simulink model "Servo_model_n"  (R2022b)
settings: Solver=ode5  StartTime=0.0  StopTime=5  FixedStep=0.01  RelTol=1e-3  AbsTol=1e-6
PreLoadFcn:
  | load servo_chstat
undefined symbols (not defined in the file or in its folder): pwm, vpwm
settings Model: ExtModeTrigDuration=12000  ExtModeTrigLevel=0.400000  Creator=jims  LastModifiedBy=artur
settings SolverCC: AutoScaleAbsTol=off  AlgebraicLoopSolver=TrustRegion
settings DataIOCC: ExternalInput=[]  InitialState=[]  MaxDataPoints=5000  SaveFormat=Array  SignalLoggingSaveFormat=ModelDataLogs  SaveOutput=off  SaveTime=off  ReturnWorkspaceOutputs=off  SignalLoggingName=sigsOut
settings OptimizationCC: BooleanDataType=off  ExpressionDepthLimit=2147483647  LifeSpan=inf
settings DebuggingCC: SaveWithParameterizedLinksMsg=none  UnderspecifiedInitializationDetection=Classic  MergeDetectMultiDrivingBlocksExec=none  SignalResolutionControl=TryResolveAllWithWarning  MultiTaskDSMMsg=warning  MultiTaskCondExecSysMsg=none  IntegerOverflowMsg=none  FcnCallInpInsideContextMsg=warning  UnconnectedInputMsg=warning  UnconnectedOutputMsg=warning  UnconnectedLineMsg=warning  AllowSymbolicDim=off  StateNameClashWarn=warning  PregeneratedLibrarySubsystemCodeDiagnostic=none  SFUnexpectedBacktrackingDiag=warning  SFNoUnconditionalDefaultTransitionDiag=warning  SFExecutionAtInitializationDiag=none  SFMachineParentedDataDiag=warning  IntegerSaturationMsg=none  ArithmeticOperatorsInVariantConditions=warning
settings HardwareCC: ProdBitPerLong=64  ProdHWDeviceType=Intel->x86-64 (Linux 64)  TargetBitPerLong=64  TargetBitPerPointer=64  TargetIntDivRoundTo=Zero  TargetEndianess=LittleEndian  TargetWordSize=64  TargetHWDeviceType=Intel->x86-64
settings ModelReferenceCC: EnableRefExpFcnMdlSchedulingChecks=on  PropagateSignalLabelsOutOfModel=off
settings SFSimCC: SimUseLocalCustomCode=off  CustomCodeUndefinedFunction=UseInterfaceOnly
settings RTWCC: Description=Simulink Desktop Real-Time  SystemTargetFile=sldrt.tlc  TemplateMakefile=sldrt.tmf  RTWUseLocalCustomCode=off  RTWCompilerOptimization=on
settings CodeAppCC: MaxIdLength=95  StateflowObjectComments=on
settings SimulinkDesktopRealTimeCC: TargetLibSuffix=_sldrt.a  TargetPreCompLibLocation=C:\Program Files\MATLAB\R2022b\toolbox\sldrt\lib\win64  TargetLangStandard=C89/C90 (ANSI)  SupportVariableSizeSignals=off
settings ConfigComp: CovMetricSettings=dw  CovSaveCumulativeToWorkspaceVar=on  CovSaveSingleToWorkspaceVar=on  CovExternalEMLEnable=off

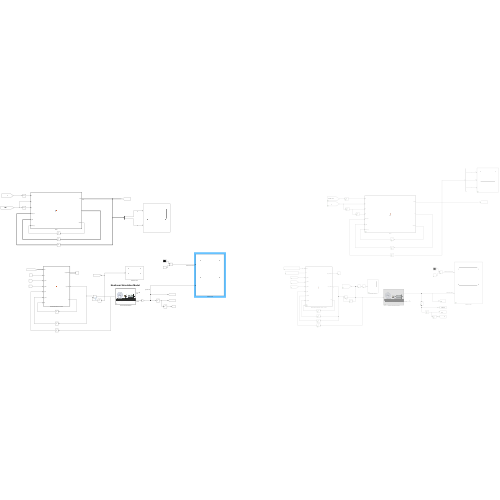
[thumbnail: Simulink's stored preview of the top-level diagram]
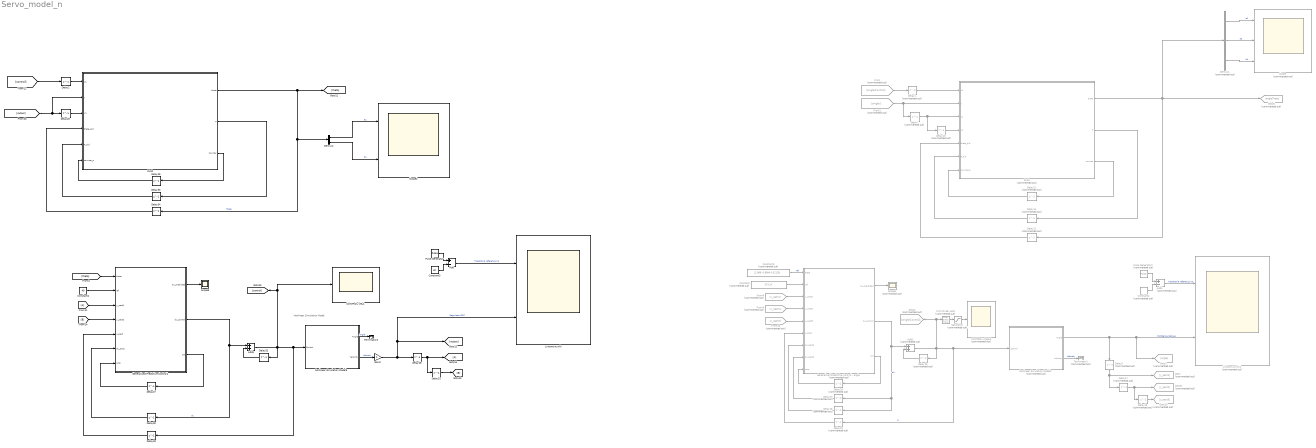
== system Servo_model_n ==
  note: Nonlinear Simulation Model
  Add : Sum  Inputs=+-
  Add2 : Sum  Commented=on
  Add3 : Sum
  Add4 : Sum  Commented=on  Inputs=+-
  CONTROL ANGLE : Scope  Commented=on
  CONTROL VEL1 : Scope
  Constant : Constant  Commented=on  Value=2*3.14
  Constant2 : Constant  Value=40
  Constant3 : Constant  Value=40
  Constant4 : Constant  Commented=on  Value=2*3.14
  Constant6 : Constant  Commented=on  Value=[1.988 -0.9884 0.01129]
  Delay1 : Delay  Commented=on  InitialCondition=0
  Delay{3,7,10,15..19} (8 alike) : Delay  Commented=on  DelayLength=1  InitialCondition=0
  Delay12 : Delay  Commented=on  DelayLength=1  InitialCondition=[2 -1 0.01]
  Delay14 : Delay  Commented=on  DelayLength=1  InitialCondition=eye(3) * 10^6
  Delay{2,25,28..32} (7 alike) : Delay  DelayLength=1  InitialCondition=0
  Delay20 : Delay  Commented=on  InitialCondition=0
  Delay21 : Delay  Commented=on  DelayLength=1  InitialCondition=10
  Delay24 : Delay  Commented=on  DelayLength=1  InitialCondition=1
  Delay26 : Delay  DelayLength=1  InitialCondition=10
  Delay27 : Delay  DelayLength=1  InitialCondition=1
  Delay33 : Delay  DelayLength=1  InitialCondition=eye(2) * 10^6
  Delay34 : Delay  DelayLength=1  InitialCondition=[0.79 1.9048]
  Demux1 : Demux  Commented=on  Outputs=3
  Demux2 : Demux  Outputs=2
  First Order Hold : FirstOrderHold  Commented=on  ErrorTolerance=inf
  From : From  Commented=on  GotoTag=angleControl
  From1 : From  Commented=on  GotoTag=angle
  From10 : From  Commented=on  GotoTag=y_past3
  From11 : From
  From8 : From  Commented=on  GotoTag=y_past1
  From9 : From  Commented=on  GotoTag=y_past2
  Gain2 : Gain
  Generalized Predictive Control - angle : MATLAB Function  Commented=on  TreatAsAtomicUnit=on
  Generalized Predictive Control1 : MATLAB Function  TreatAsAtomicUnit=on
  Goto : Goto  Commented=on  GotoTag=y_past1
  Goto1 : Goto  Commented=on  GotoTag=angle
  Goto10 : Goto  Commented=on  GotoTag=y_past3
  Goto14 : Goto
  Goto2 : Goto  Commented=on  GotoTag=angleControl
  Goto5 : Goto  Commented=on  GotoTag=angleTheta
  Goto9 : Goto  Commented=on  GotoTag=y_past2
  Liniowe wyniki : Scope  NumInputPorts=2
  Liniowe wyniki1 : Scope  Commented=on  NumInputPorts=2
  Nonlinear Simulation Model2 : Subsystem  Commented=on  mask{x0=[0 0], c_n=206, Parameter3=[vpwm pwm]}
      mask prompts: x0 "Initial conditions [angle velocity]"; c_n "Gain c"; Parameter3 "Static characteristic [velocity control]"
      mask Help:
      | The parameters necessary for this block are:
      | 1. Static characteristic implemented as Look-up table block (vectors vpwm and pwm),
      | 2. gain  - c ,
      | 3. Initial conditions - x0,
      | Refer to 3.2 section in User's Manual.
      | 
      | 
      | The model preloads the default static characteristic from servo_chstat.mat file.
      | To change default characteristic a user should load a new vpwm and pwm vectors or
      | replace servo_chstat.mat file.
      mask Display: image(imread('Servo_m.JPG'))
  Nonlinear Simulation Model3 : Subsystem  mask{x0=[0 0], c_n=206, Parameter3=[vpwm pwm]}
      mask prompts: x0 "Initial conditions [angle velocity]"; c_n "Gain c"; Parameter3 "Static characteristic [velocity control]"
      mask Help:
      | The parameters necessary for this block are:
      | 1. Static characteristic implemented as Look-up table block (vectors vpwm and pwm),
      | 2. gain  - c ,
      | 3. Initial conditions - x0,
      | Refer to 3.2 section in User's Manual.
      | 
      | 
      | The model preloads the default static characteristic from servo_chstat.mat file.
      | To change default characteristic a user should load a new vpwm and pwm vectors or
      | replace servo_chstat.mat file.
      mask Display: image(imread('Servo_m.JPG'))
  Pulse Generator : DiscretePulseGenerator  PulseType=Time based  Amplitude=80  Period=4  PulseWidth=50
  Pulse Generator2 : DiscretePulseGenerator  Commented=on  PulseType=Time based  Amplitude=4*pi  Period=4  PulseWidth=50
  RLS1 : MATLAB Function  Commented=on  TreatAsAtomicUnit=on
  RLS2 : MATLAB Function  TreatAsAtomicUnit=on
  Saturation : Saturate  Commented=on  UpperLimit=1  LowerLimit=-1
  Scope : Scope  Commented=on  NumInputPorts=3
  Scope2 : Scope  NumInputPorts=2
  Scope4 : Scope  Commented=on
  Scope5 : Scope
  Terminator1 : Terminator  Commented=on
  Terminator2 : Terminator
  wires:
  Gain2/1 -> Delay28/1, [output], Liniowe wyniki/2  "Regulator GPC"
  Delay30/1 -> Generalized Predictive Control1/6(du_past)
  [control] -> Delay2/1
  RLS2/1(theta) -> Demux2/1, Delay34/1, [theta]  "theta"
  Generalized Predictive Control1/1(du_predicted) -> Scope5/1
  Delay34/1 -> RLS2/4(theta_old)
  Delay33/1 -> RLS2/5(P_old)
  [output] -> Delay25/1, RLS2/2(y)
  Nonlinear Simulation Model3/1(Angle) -> Terminator2/1  "Angle"
  Demux2/2 -> Scope2/2  "b1"
  Nonlinear Simulation Model3/2(Velocity) -> Gain2/1  "Velocity"
  [B] -> Generalized Predictive Control1/4(y_past2)
  [theta] -> Generalized Predictive Control1/1(theta)
  Delay28/1 -> Delay31/1, Goto14/1
  Delay25/1 -> RLS2/3(y1)
  Add3/1 -> CONTROL VEL1/1, [control], Nonlinear Simulation Model3/1(Control), Delay29/1, Delay32/1
  From11/1 -> Generalized Predictive Control1/3(y_past1)
  Delay26/1 -> RLS2/6(counter_p)
  Delay29/1 -> Generalized Predictive Control1/5(u_past)
  Constant3/1 -> Add/2
  Constant2/1 -> Generalized Predictive Control1/2(ref)
  Pulse Generator/1 -> Add/1
  Generalized Predictive Control1/3(cnt) -> Delay27/1
  Add/1 -> Liniowe wyniki/1  "Trajektoria referencyjna"
  Delay32/1 -> Add3/2
  Delay27/1 -> Generalized Predictive Control1/7(cntp)
  RLS2/3(counter) -> Delay26/1
  Delay2/1 -> RLS2/1(u1)
  Generalized Predictive Control1/2(du_control) -> Delay30/1, Add3/1  "du"
  Delay31/1 -> [B]
  Demux2/1 -> Scope2/1  "a1"
  RLS2/2(P) -> Delay33/1
  From9/1 -> Generalized Predictive Control - angle/4(y_past2)
  From10/1 -> Generalized Predictive Control - angle/5(y_past3)
  Constant4/1 -> Add4/2
  Nonlinear Simulation Model2/1(Angle) -> Delay3/1, Liniowe wyniki1/2, Goto1/1  "Położenie kątowe"
  RLS1/1(theta) -> Delay12/1, Goto5/1, Demux1/1
  Delay3/1 -> Delay17/1, Goto/1
  Saturation/1 -> CONTROL ANGLE/1
  First Order Hold/1 -> Saturation/1
  Generalized Predictive Control - angle/3(cnt) -> Delay24/1
  Delay18/1 -> Goto10/1
  Delay19/1 -> Generalized Predictive Control - angle/6(u_past)
  Delay21/1 -> RLS1/7(counter_p)
  RLS1/3(counter) -> Delay21/1
  Pulse Generator2/1 -> Add4/1
  Generalized Predictive Control - angle/2(du_control) -> Delay16/1, Delay20/1, Add2/1  "du"
  Constant/1 -> Generalized Predictive Control - angle/2(ref)
  Constant6/1 -> Generalized Predictive Control - angle/1(theta)  "ref"
  From1/1 -> Delay7/1, RLS1/2(y)
  Delay24/1 -> Generalized Predictive Control - angle/9(cntp)
  From8/1 -> Generalized Predictive Control - angle/3(y_past1)
  Demux1/2 -> Scope/2  "a2"
  Demux1/3 -> Scope/3  "b1"
  Nonlinear Simulation Model2/2(Velocity) -> Terminator1/1  "Velocity"
  Add4/1 -> Liniowe wyniki1/1  "Trajektoria referencyjna"
  RLS1/2(P) -> Delay14/1
  Delay15/1 -> Add2/2
  Delay10/1 -> RLS1/4(y2)
  Generalized Predictive Control - angle/1(du_predicted) -> Scope4/1
  Delay16/1 -> Generalized Predictive Control - angle/7(du_past1)
  Delay14/1 -> RLS1/6(P_old)
  Delay7/1 -> Delay10/1, RLS1/3(y1)
  From/1 -> Delay1/1
  Delay1/1 -> RLS1/1(u2)
  Delay12/1 -> RLS1/5(theta_old)
  Add2/1 -> First Order Hold/1, Goto2/1, Delay15/1, Nonlinear Simulation Model2/1(Control), Delay19/1  "S"
  Delay17/1 -> Delay18/1, Goto9/1
  Delay20/1 -> Generalized Predictive Control - angle/8(du_past2)
  Demux1/1 -> Scope/1  "a1"

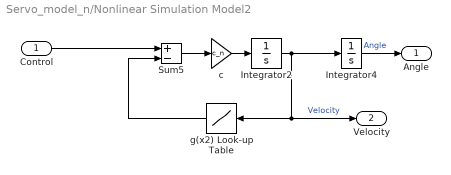
== system Servo_model_n/Nonlinear Simulation Model2 ==
  Control : Inport
  Integrator2 : Integrator  InitialCondition=x0(2)
  Integrator4 : Integrator  InitialCondition=x0(1)
  Sum5 : Sum  Inputs=+-  InputSameDT=on  SaturateOnIntegerOverflow=on  OutDataTypeStr=Inherit: Same as first input
  c : Gain  Gain=c_n  SaturateOnIntegerOverflow=on  OutDataTypeStr=Inherit: Same as input  ParamDataTypeStr=Inherit: Same as input
  g(x2) Look-up Table : Lookup  InputValues=vpwm  Table=pwm
  Angle : Outport  InitialOutput=0  VectorParamsAs1DForOutWhenUnconnected=off
  Velocity : Outport  Port=2  InitialOutput=0  VectorParamsAs1DForOutWhenUnconnected=off
  wires:
  Control/1 -> Sum5/1
  c/1 -> Integrator2/1
  Integrator4/1 -> Angle/1  "Angle"
  Integrator2/1 -> g(x2) Look-up Table/1, Velocity/1, Integrator4/1  "Velocity"
  g(x2) Look-up Table/1 -> Sum5/2
  Sum5/1 -> c/1

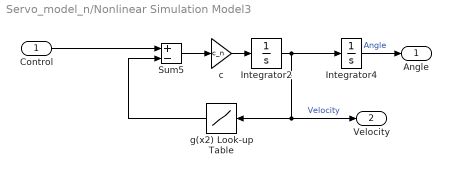
== system Servo_model_n/Nonlinear Simulation Model3 ==
  Control : Inport
  Integrator2 : Integrator  InitialCondition=x0(2)
  Integrator4 : Integrator  InitialCondition=x0(1)
  Sum5 : Sum  Inputs=+-  InputSameDT=on  SaturateOnIntegerOverflow=on  OutDataTypeStr=Inherit: Same as first input
  c : Gain  Gain=c_n  SaturateOnIntegerOverflow=on  OutDataTypeStr=Inherit: Same as input  ParamDataTypeStr=Inherit: Same as input
  g(x2) Look-up Table : Lookup  InputValues=vpwm  Table=pwm
  Angle : Outport  InitialOutput=0  VectorParamsAs1DForOutWhenUnconnected=off
  Velocity : Outport  Port=2  InitialOutput=0  VectorParamsAs1DForOutWhenUnconnected=off
  wires:
  Control/1 -> Sum5/1
  c/1 -> Integrator2/1
  Integrator4/1 -> Angle/1  "Angle"
  Integrator2/1 -> g(x2) Look-up Table/1, Velocity/1, Integrator4/1  "Velocity"
  g(x2) Look-up Table/1 -> Sum5/2
  Sum5/1 -> c/1

== matlab function Servo_model_n/RLS1 ==
  data: u2 input; y input; y1 input; y2 input; theta output; theta_old input; P_old input; P output; counter_p input; counter output
function [theta,P,counter]= fcn(u2,y,y1,y2,theta_old,P_old,counter_p)

counter = counter_p;

lambda = 0.985;

phi = [y1;y2;u2];

if counter_p == 10

K = P_old * phi/(lambda + phi'*P_old*phi);

P = ((eye(3) - K * phi') * P_old) * lambda^-1;

theta = theta_old + K * (y - phi'*theta_old);

counter = 0;
else

theta = theta_old;
P = P_old;
counter = counter + 1;
end

== matlab function Servo_model_n/Generalized Predictive Control - angle ==
  data: du_predicted output; theta input; ref input; y_past1 input; y_past2 input; y_past3 input; u_past input; du_past1 input; du_control output; du_past2 input; cnt output; cntp input
function [du_predicted, du_control,cnt] = fcn(theta,ref,y_past1,y_past2,y_past3,u_past,du_past1,du_past2,cntp)

cnt = cntp;

%Współczynniki modelu z algorytmu RLS
a1 = -theta(1);
a2 = -theta(2);
b1 = theta(3);

%Parametry
ny = 32; %HORYZONT PREDYKCJI
nu = 8; %HORYZONT STEROWANIA
lambda = 1.2;

%Przeszłe wyjścia
y_past = [y_past1;y_past2;y_past3];
du_past = [du_past1;du_past2];

%Trajektoria referencyjna, stała

%%% trajektoria referencyjna
Ts = 0.01; %PRÓBKOWANIE SYMULACJI
sim_time = 4; %CZAS SYMULACJI

traj_ub = ref*ones(1/Ts*sim_time/2,1);

traj_lb = -ref*ones(1/Ts*sim_time/2,1);


trajektoria = [traj_ub;traj_lb;traj_ub];

ref = trajektoria(cnt:ny+cnt-1, 1);

cnt = cntp + 1;

if cnt == 30*100-ny
    cnt = 1;
end

%%%

%Czy wykorzystać T-filtr?
filtrowanie = false;

%Ograniczenia
%true - ograniczenia na y, false - bez ograniczeń na y
ograniczenie_wyjscia = true;

du_max = 1;
du_min = -1;
u_max = 1;
u_min = -1;
y_max = 6.6;
y_min = -6.6;

%Wyznaczenie wielomianów a i b
a = [1 a1 a2];
b = [0 0 b1];
A = conv(a,[1 -1]);

%Wyznaczenie macierzy predykcji
[Ca,Ha] = predmat(A,ny);
[Cb,Hb] = predmat(b,ny);

Cai = inv(Ca);

H = Cai*Cb;
P = Cai*Hb;
Q = Cai*(-Ha);

%%%%%%%%%%%%%%%%%%%%%%%%%%%%%%%%%%%%%%%%%%%%%%%%%%%%%%%%%%%%%%%%%%%%%%%%%%%

if filtrowanie == true
    Tfilt = [1 -0.05];
    
    [Ct,Ht] = predmat(Tfilt,ny);
    Pfilt = Ct * P - H * Ht;
    Qfilt = Ct * Q + Ht;
    
    P = Pfilt;
    Q = Qfilt;
end

%%%%%%%%%%%%%%%%%%%%%%%%%%%%%%%%%%%%%%%%%%%%%%%%%%%%%%%%%%%%%%%%%%%%%%%%%%%

Hu = H(:,1:nu); %horyzont sterowania

%Ustawienie ograniczeń dla optymalizatora 

%Prawo sterowania dla algorytmu z ograniczeniami
S = Hu'*Hu + eye(nu)*lambda;
S = (S + S')/2;
f = Hu'*Q * y_past + Hu'*P * du_past - Hu' * ref;

    if ograniczenie_wyjscia == true
        %OGRANICZENIA Z Y
        [C,dd,du,ddu,dy] = mpc_ograniczenia(du_max, du_min,u_max,u_min,y_max,y_min,nu,Hu,P,Q,2,3);
        dt = dd + du * u_past + ddu * du_past + dy*y_past;
    else
        %OGRANICZENIA BEZ Y
        [C, dd,du] = mpc_ograniczenia_bez_y(du_max,du_min,u_max,u_min,nu);
        dt = dd + du * u_past;
    end


opts = optimoptions('quadprog','Algorithm','active-set');

x0 = 0.1*eye(nu,1);

du_predicted = quadprog(S,f,C,dt,[],[],[],[],x0,opts);

du_control = du_predicted(1);

%Prawo sterowania dla algorytmu bez ograniczeń
% Pr = ( inv(Hu'*Hu+lambda*eye(nu)) ) * Hu';
% Nk = Pr*Q;
% Dk = Pr*P;
% 
% du_predicted = Pr * ref - Dk * du_past - Nk*y_past;
% du_control = du_predicted(1);

== matlab function Servo_model_n/Generalized Predictive Control1 ==
  data: du_predicted output; theta input; ref input; y_past1 input; y_past2 input; u_past input; du_past input; du_control output; cntp input; cnt output
function [du_predicted, du_control,cnt] = fcn(theta,ref,y_past1,y_past2,u_past,du_past,cntp)

cnt = cntp;

%Współczynniki modelu z algorytmu RLS
a1 = -theta(1);
b1 = theta(2);

%Przeszłe wyjścia
y_past = [y_past1;y_past2];
    
%Parametry
ny = 32; %HORYZONT PREDYKCJI
nu = 12; %HORYZONT STEROWANIA
lambda = 0.5;
    
%Czy wykorzystać T-filtr?
filtrowanie = false;
    
%Ograniczenia
%true - ograniczenia na y, false - bez ograniczeń na y
ograniczenie_wyjscia = true;

du_max = 1;
du_min = -1;
u_max = 1;
u_min = -1;
y_max = 42;
y_min = -42;

%Trajektoria referencyjna, stała
Ts = 0.01; %PRÓBKOWANIE SYMULACJI
sim_time = 4; %CZAS SYMULACJI

traj_ub = ref*ones(1/Ts*sim_time/2,1);

traj_lb = -ref*ones(1/Ts*sim_time/2,1);

%%% trajektoria referencyjna
trajektoria = [traj_ub;traj_lb;traj_ub;-ref*ones(ny,1)];

ref = trajektoria(cnt:ny+cnt-1, 1);

cnt = cntp + 1;

%%%



    %Wyznaczenie wielomianów a i b
    a = [1 a1];
    b = [0 b1];
    A = conv(a,[1 -1]);
    
    %Wyznaczenie macierzy predykcji
    [Ca,Ha] = predmat(A,ny);
    [Cb,Hb] = predmat(b,ny);
    
    Cai = inv(Ca);
    
    H = Cai*Cb;
    P = Cai*Hb;
    Q = Cai*(-Ha);

%%%%%%%%%%%%%%%%%%%%%%%%%%%%%%%%%%%%%%%%%%%%%%%%%%%%%%%%%%%%%%%%%%%%%%%%%%%

if filtrowanie == true
    Tfilt = [1 -0.2];
    
    [Ct,Ht] = predmat(Tfilt,ny);
    Pfilt = Ct * P - H * Ht;
    Qfilt = Ct * Q + Ht;
    
    P = Pfilt;
    Q = Qfilt;
end

%%%%%%%%%%%%%%%%%%%%%%%%%%%%%%%%%%%%%%%%%%%%%%%%%%%%%%%%%%%%%%%%%%%%%%%%%%%

    Hu = H(:,1:nu); %horyzont sterowania

%Ustawienie ograniczeń dla optymalizatora 

%Prawo sterowania dla algorytmu z ograniczeniami
    S = Hu'*Hu + eye(nu)*lambda;
    S = (S + S')/2;
    f = Hu'*Q * y_past + Hu'*P * du_past - Hu' * ref;

    if ograniczenie_wyjscia == true
        %OGRANICZENIA Z Y
        [C,dd,du,ddu,dy] = mpc_ograniczenia(du_max, du_min,u_max,u_min,y_max,y_min,nu,Hu,P,Q,1,2);
        dt = dd + du * u_past + ddu * du_past + dy*y_past;
    else
        %OGRANICZENIA BEZ Y
        [C, dd,du] = mpc_ograniczenia_bez_y(du_max,du_min,u_max,u_min,nu);
        dt = dd + du * u_past;
    end


    opts = optimoptions('quadprog','Algorithm','active-set');

    x0 = 0.1*eye(nu,1);

    du_predicted = quadprog(S,f,C,dt,[],[],[],[],x0,opts);

    du_control = du_predicted(1);


%Prawo sterowania dla algorytmu bez ograniczeń
% Pr = ( inv(Hu'*Hu+lambda*eye(nu)) ) * Hu';
% Nk = Pr*Q;
% Dk = Pr*P;
% 
% du_predicted = Pr * ref - Dk * du_past - Nk*y_past;
% du_control = du_predicted(1);

== matlab function Servo_model_n/RLS2 ==
  data: u1 input; y input; y1 input; theta output; theta_old input; P_old input; P output; counter_p input; counter output
function [theta,P,counter]= fcn(u1,y,y1,theta_old,P_old,counter_p)

counter = counter_p;

if counter_p == 10

lambda = 0.985;
phi = [y1;u1];

K = P_old * phi/(lambda + phi'*P_old*phi);

P = ((eye(2) - K * phi') * P_old) * lambda^-1;

theta = theta_old + K * (y - phi'*theta_old);

counter = 1;
else
    theta = theta_old;
    P = P_old;
    counter = counter + 1;
end
